simulink subsystem "drgkbh"  (R2022b)
settings: Solver=VariableStepAuto  StartTime=0.0  StopTime=10.0  RelTol=1e-3
settings Model: Creator=EDKI  LastModifiedBy=EDKI

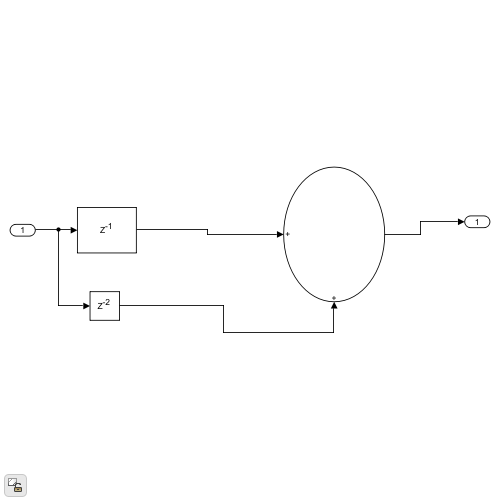
[thumbnail: Simulink's stored preview of the top-level diagram]
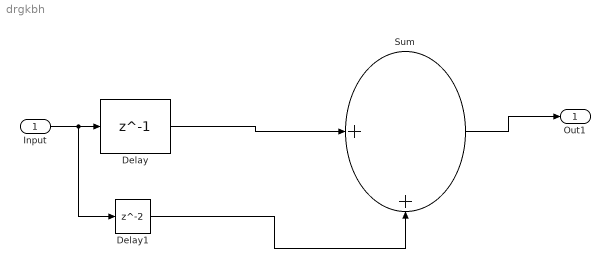
== system drgkbh ==
  Input : Inport
  Delay : Delay  DelayLength=1
  Delay1 : Delay
  Sum : Sum  Inputs=|++
  Out1 : Outport
  wires:
  Sum/1 -> Out1/1
  Delay/1 -> Sum/1
  Delay1/1 -> Sum/2
  Input/1 -> Delay1/1, Delay/1
